simulink model "kinematic_model"  (R2022b)
settings: Solver=FixedStepAuto  StartTime=0.0  StopTime=10.0  FixedStep=0.01  RelTol=1e-3
values from neighbouring files (symbols this model uses):
  IC_theta0 = 0    [ModelConstants.mat]
  IC_theta1 = 0    [ModelConstants.mat]
  IC_x0 = 0    [ModelConstants.mat]
  IC_y0 = 0    [ModelConstants.mat]
  L_0b = 0.3    [ModelConstants.mat]
  L_0f = 3.8    [ModelConstants.mat]
  L_1f = 8.475    [ModelConstants.mat]
settings Model: Creator=makannan  LastModifiedBy=makannan

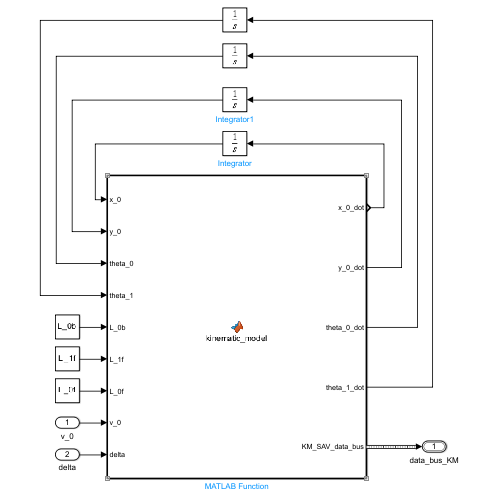
[thumbnail: Simulink's stored preview of the top-level diagram]
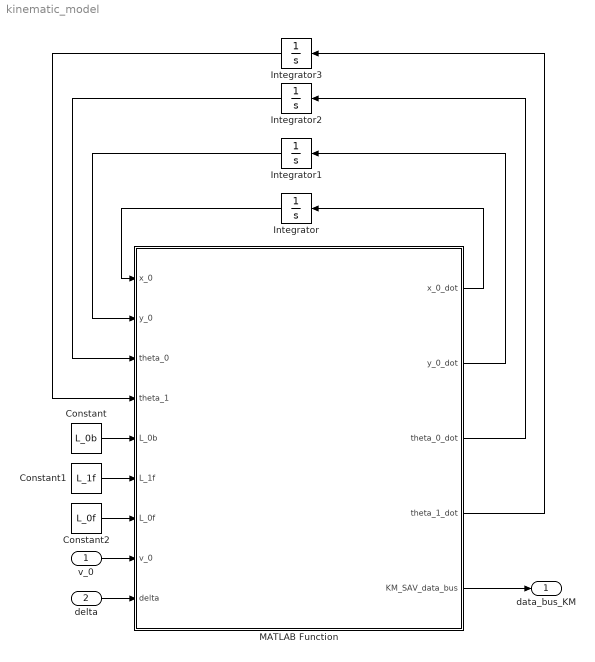
== system kinematic_model ==
  v_0 : Inport
  delta : Inport  Port=2
  Constant : Constant  Value=L_0b
  Constant1 : Constant  Value=L_1f
  Constant2 : Constant  Value=L_0f
  Integrator : Integrator  InitialCondition=IC_x0
  Integrator1 : Integrator  InitialCondition=IC_y0
  Integrator2 : Integrator  InitialCondition=IC_theta0
  Integrator3 : Integrator  InitialCondition=IC_theta1
  MATLAB Function : MATLAB Function  TreatAsAtomicUnit=on
  data_bus_KM : Outport  OutDataTypeStr=Bus: data_bus_KM
  wires:
  MATLAB Function/1(x_0_dot) -> Integrator/1
  Integrator/1 -> MATLAB Function/1(x_0)
  MATLAB Function/2(y_0_dot) -> Integrator1/1
  Integrator1/1 -> MATLAB Function/2(y_0)
  MATLAB Function/3(theta_0_dot) -> Integrator2/1
  Integrator2/1 -> MATLAB Function/3(theta_0)
  MATLAB Function/4(theta_1_dot) -> Integrator3/1
  Integrator3/1 -> MATLAB Function/4(theta_1)
  Constant/1 -> MATLAB Function/5(L_0b)
  Constant1/1 -> MATLAB Function/6(L_1f)
  Constant2/1 -> MATLAB Function/7(L_0f)
  v_0/1 -> MATLAB Function/8(v_0)
  delta/1 -> MATLAB Function/9(delta)
  MATLAB Function/5(KM_SAV_data_bus) -> data_bus_KM/1

== matlab function kinematic_model/MATLAB Function ==
  data: x_0 input; x_0_dot output; y_0 input; theta_0 input; theta_1 input; L_0b input; L_1f input; L_0f input; v_0 input; delta input; y_0_dot output; theta_0_dot output; theta_1_dot output; KM_SAV_data_bus output Bus: data_bus_KM
function [x_0_dot,y_0_dot,theta_0_dot,theta_1_dot,KM_SAV_data_bus] = kinematic_model(x_0,y_0,theta_0,theta_1,L_0b,L_1f,L_0f,v_0,delta)


[x_0_dot,y_0_dot,theta_0_dot,theta_1_dot,KM_SAV_data_bus] = vehicle.kinematic_model(x_0,y_0,theta_0,theta_1,L_0b,L_1f,L_0f,v_0,delta);
